simulink model "ODE_Hand_Model_v01_faulty"  (Simulink 7.5)
settings: Solver=ode1  StartTime=0.0  StopTime=inf  FixedStep=0.0315/3  RelTol=1e-3
settings Model: Creator=nihil  LastModifiedBy=konstantinos

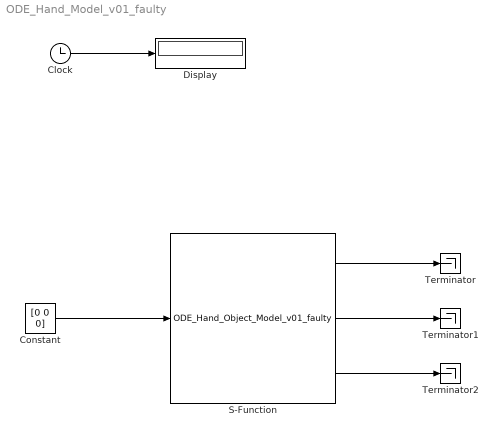
== system ODE_Hand_Model_v01_faulty ==
  Clock : Clock
      settings: Decimation=10
  Constant : Constant  Value=[0 0 0]  OutDataType=fixdt(1, 16)  OutScaling=2^0
  Display : Display
  S-Function : S-Function  FunctionName=ODE_Hand_Object_Model_v01_faulty  EnableBusSupport=off
  Terminator : Terminator
  Terminator1 : Terminator
  Terminator2 : Terminator
  wires:
  Clock/1 -> Display/1
  Constant/1 -> S-Function/1
  S-Function/1 -> Terminator/1
  S-Function/2 -> Terminator1/1
  S-Function/3 -> Terminator2/1
